simulink model "main"  (R2025a)
settings: Solver=FixedStepAuto  StartTime=0.0  StopTime=20  FixedStep=0.005  RelTol=1e-3
model workspace (MAT data in the model file):
  lowerLimit = 25
  speedMax = 10
  upperLimit = 75
libraries: simulink x5, simulink_extras x2
settings Model: PacingRate=0.100000  ParameterArgumentNames=speedMax  LastModifiedBy=alexc
settings SolverCC: ZeroCrossAlgorithm=Adaptive
settings OptimizationCC: BlockReduction=off  DefaultParameterBehavior=Inlined  BufferReuse=off
settings DebuggingCC: IgnoredZcDiagnostic=none
settings RTWCC: GPUComputeCapability=3.5

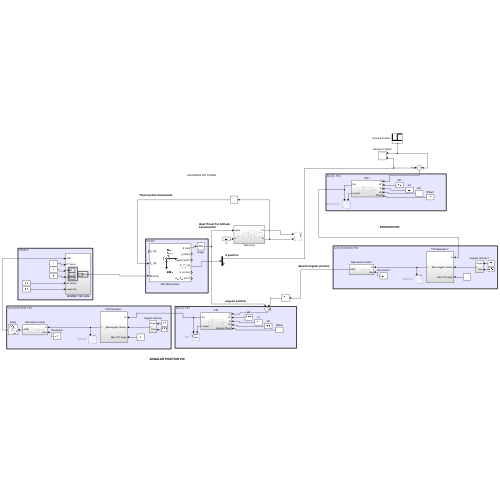
[thumbnail: Simulink's stored preview of the top-level diagram]
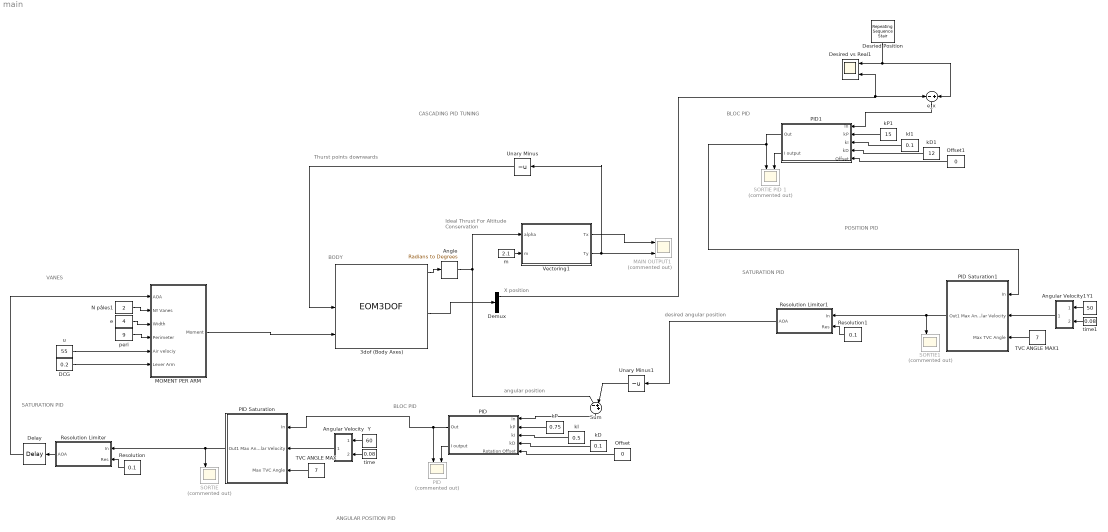
== system main ==
  note: CASCADING PID TUNING
  note: VANES
  note: SATURATION PID
  note: BODY
  note: BLOC PID
  note: BLOC PID
  note: SATURATION PID
  note: ANGULAR POSITION PID
  note: POSITION PID
  note: desired angular position
  note: angular position
  note: X position
  note: Ideal Thrust For Altitude Conservation
  note: Thurst points downwards
  3dof (Body Axes) : EOM3DOF  v_ini=0.0  mass=2.1  Iyy=0.038
  Angle : simulink_extras/Transformations/Radians to Degrees
  Angular Velocity : Subsystem
  Angular Velocity1 : Subsystem
  DCG : Constant  Value=0.2
  Delay : TransportDelay  DelayTime=0.005
  Demux : Demux  Outputs=2
  Desired vs Real1 : Scope  NumInputPorts=2
      settings: ActiveDisplayYMinimum=-0.47513093423326325  ActiveDisplayYMaximum=1.2413964602453749  DataLoggingVariableName=ScopeData5
  Desried Position : simulink/Sources/Repeating Sequence Stair  OutValues=[0,0.5]  tsamp=5  OutMin=[]  OutMax=[]  OutDataTypeStr=double  OutputDataTypeScalingMode=double  OutDataType=fixdt(0,8)  ConRadixGroup=Best Precision: Vector-wise  OutScaling=2^-12
  MAIN OUTPUT1 : Scope  Commented=on  NumInputPorts=2
      settings: ActiveDisplayYMinimum=-7.2954565061665075  ActiveDisplayYMaximum=8.1972905138472143
  MOMENT PER ARM : Subsystem
  N pâles1 : Constant  Value=2
  Offset : Constant  Value=0
  Offset1 : Constant  Value=0
  PID : Subsystem
  "PID " : Scope  Commented=on  NumInputPorts=2
      settings: ActiveDisplayYMinimum=-1  ActiveDisplayYMaximum=1  DataLoggingVariableName=ScopeData2
  PID Saturation : Subsystem
  PID Saturation1 : Subsystem
  PID1 : Subsystem
  Resolution : Constant  Value=0.1
  Resolution Limiter : Subsystem
  Resolution Limiter1 : Subsystem
  Resolution1 : Constant  Value=0.1
  SORTIE : Scope  Commented=on  NumInputPorts=2
      settings: ActiveDisplayYMinimum=-4.7113055005925766  ActiveDisplayYMaximum=4.7400570614554063  DataLoggingVariableName=ScopeData3
  SORTIE PID 1 : Scope  Commented=on  NumInputPorts=2
      settings: ActiveDisplayYMinimum=-12.890019352099706  ActiveDisplayYMaximum=16.05060564784133  DataLoggingVariableName=ScopeData4
  SORTIE1 : Scope  Commented=on  NumInputPorts=2
      settings: ActiveDisplayYMinimum=-6.75  ActiveDisplayYMaximum=0.75  DataLoggingVariableName=ScopeData6
  Sum : Sum  Inputs=|-++
  TVC ANGLE MAX : Constant  Value=7
  TVC ANGLE MAX1 : Constant  Value=7
  Unary Minus : UnaryMinus
  Unary Minus1 : UnaryMinus
  Vectoring1 : Subsystem
  Y : Constant  Value=60
  Y1 : Constant  Value=50
  e : Constant  Value=4
  e_x : Sum  Inputs=-+
  kD : Constant  Value=0.1
  kD1 : Constant  Value=12
  kI : Constant  Value=0.5
  kI1 : Constant  Value=0.1
  kP : Constant  Value=0.75
  kP1 : Constant  Value=15
  m : Constant  Value=2.1
  peri : Constant  Value=9
  time : Constant  Value=0.08
  time1 : Constant  Value=0.08
  u : Constant  Value=55
  wires:
  Angle/1 -> Sum/1, Vectoring1/1(alpha)
  3dof (Body Axes)/1 -> Angle/1
  N pâles1/1 -> MOMENT PER ARM/2(Nº Vanes)
  DCG/1 -> MOMENT PER ARM/6(Lever Arm)
  u/1 -> MOMENT PER ARM/5(Air velociy)
  e/1 -> MOMENT PER ARM/3(Width)
  peri/1 -> MOMENT PER ARM/4(Perimeter)
  Sum/1 -> PID/1(In)
  kP/1 -> PID/2(kP)
  kI/1 -> PID/3(kI)
  kD/1 -> PID/4(kD)
  Angular Velocity/1(Out1) -> PID Saturation/2(Max Angular Velocity)
  Y/1 -> Angular Velocity/1(Angle)
  time/1 -> Angular Velocity/2(Time)
  PID Saturation/1(Out1) -> Resolution Limiter/1(In), SORTIE/1
  Resolution/1 -> Resolution Limiter/2(Res)
  PID/1(Out) -> PID Saturation/1(In), "PID "/1
  TVC ANGLE MAX/1 -> PID Saturation/3(Max TVC Angle)
  Resolution Limiter/1(AOA) -> Delay/1
  Offset/1 -> PID/5(Rotation Offset)
  PID/2(I output) -> "PID "/2
  Delay/1 -> MOMENT PER ARM/1(AOA)
  MOMENT PER ARM/1(Moment) -> 3dof (Body Axes)/3
  m/1 -> Vectoring1/2(m)
  Vectoring1/2(Ty) -> Unary Minus/1, MAIN OUTPUT1/2
  Vectoring1/1(Tx) -> MAIN OUTPUT1/1
  3dof (Body Axes)/4 -> Demux/1
  Unary Minus/1 -> 3dof (Body Axes)/2
  Desried Position/1 -> e_x/2, Desired vs Real1/1
  PID1/2(I output) -> SORTIE PID 1/2
  e_x/1 -> PID1/1(In)
  kP1/1 -> PID1/2(kP)
  Offset1/1 -> PID1/5(Offset)
  kI1/1 -> PID1/3(kI)
  kD1/1 -> PID1/4(kD)
  time1/1 -> Angular Velocity1/2(Time)
  Y1/1 -> Angular Velocity1/1(Angle)
  PID1/1(Out) -> PID Saturation1/1(In), SORTIE PID 1/1
  TVC ANGLE MAX1/1 -> PID Saturation1/3(Max TVC Angle)
  PID Saturation1/1(Out1) -> Resolution Limiter1/1(In), SORTIE1/1
  Angular Velocity1/1(Out1) -> PID Saturation1/2(Max Angular Velocity)
  Resolution1/1 -> Resolution Limiter1/2(Res)
  Resolution Limiter1/1(AOA) -> Unary Minus1/1
  Demux/1 -> Desired vs Real1/2, e_x/1
  Unary Minus1/1 -> Sum/2

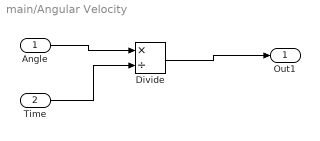
== system main/Angular Velocity ==
  Angle : Inport
  Time : Inport  Port=2
  Divide : Product  Inputs=*/
  Out1 : Outport
  wires:
  Time/1 -> Divide/2
  Angle/1 -> Divide/1
  Divide/1 -> Out1/1

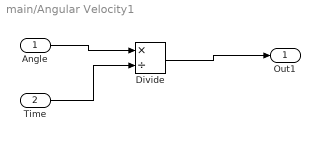
== system main/Angular Velocity1 ==
  Angle : Inport
  Time : Inport  Port=2
  Divide : Product  Inputs=*/
  Out1 : Outport
  wires:
  Time/1 -> Divide/2
  Angle/1 -> Divide/1
  Divide/1 -> Out1/1

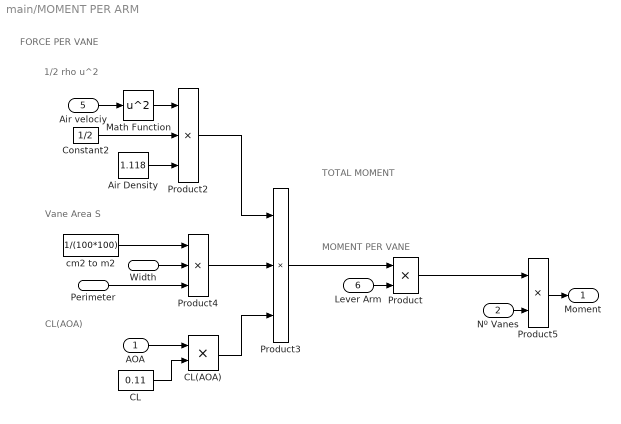
== system main/MOMENT PER ARM ==
  note: FORCE PER VANE
  note: CL(AOA)
  note: 1/2 rho u^2
  note: Vane Area S
  note: MOMENT PER VANE
  note: TOTAL MOMENT
  AOA : Inport
  Nº Vanes : Inport  Port=2
  Width : Inport  Port=3
  Perimeter : Inport  Port=4
  Air velociy : Inport  Port=5
  Lever Arm : Inport  Port=6
  Air Density : Constant  Value=1.118
  CL : Constant  Value=0.11
  CL(AOA) : Product
  Constant2 : Constant  Value=1/2
  Math Function : Math  Operator=square
  Product : Product
  Product2 : Product  Inputs=3
  Product3 : Product  Inputs=3
  Product4 : Product  Inputs=3
  Product5 : Product
  cm2 to m2 : Constant  Value=1/(100*100)
  Moment : Outport
  wires:
  Width/1 -> Product4/2
  Air velociy/1 -> Math Function/1
  cm2 to m2/1 -> Product4/1
  CL/1 -> CL(AOA)/2
  AOA/1 -> CL(AOA)/1
  Perimeter/1 -> Product4/3
  Lever Arm/1 -> Product/2
  Air Density/1 -> Product2/3
  Math Function/1 -> Product2/1
  Constant2/1 -> Product2/2
  Product/1 -> Product5/1
  Nº Vanes/1 -> Product5/2
  CL(AOA)/1 -> Product3/3
  Product4/1 -> Product3/2
  Product2/1 -> Product3/1
  Product3/1 -> Product/1
  Product5/1 -> Moment/1

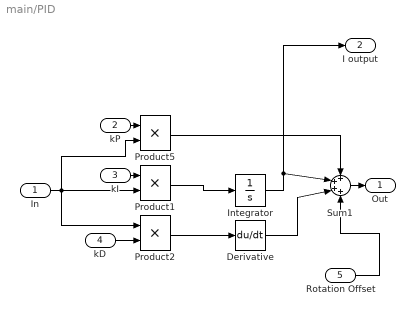
== system main/PID ==
  In : Inport
  kP : Inport  Port=2
  kI : Inport  Port=3
  kD : Inport  Port=4
  Rotation Offset : Inport  Port=5
  Derivative : Derivative
  Integrator : Integrator
  Product1 : Product
  Product2 : Product
  Product5 : Product
  Sum1 : Sum  Inputs=++++
  Out : Outport
  I output : Outport  Port=2
  wires:
  Product1/1 -> Integrator/1
  kD/1 -> Product2/2
  kI/1 -> Product1/1
  kP/1 -> Product5/1
  In/1 -> Product5/2, Product1/2, Product2/1
  Product2/1 -> Derivative/1
  Derivative/1 -> Sum1/3
  Integrator/1 -> I output/1, Sum1/2
  Product5/1 -> Sum1/1
  Sum1/1 -> Out/1
  Rotation Offset/1 -> Sum1/4

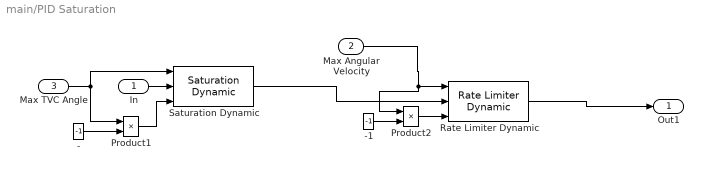
== system main/PID Saturation ==
  In : Inport
  Max Angular Velocity : Inport  Port=2
  Max TVC Angle : Inport  Port=3
  - : Constant  Value=-1
  -1 : Constant  Value=-1
  Product1 : Product
  Product2 : Product
  Rate Limiter Dynamic : simulink/Discontinuities/Rate Limiter Dynamic
  Saturation Dynamic : simulink/Discontinuities/Saturation Dynamic  OutMin=[]  OutMax=[]  OutDataTypeStr=Inherit: Same as second input  OutDataType=fixdt(1, 16)  OutScaling=2^-10  DoSatur=off
  Out1 : Outport
  wires:
  Max TVC Angle/1 -> Saturation Dynamic/1, Product1/1
  -/1 -> Product1/2
  In/1 -> Saturation Dynamic/2
  Product1/1 -> Saturation Dynamic/3
  Saturation Dynamic/1 -> Rate Limiter Dynamic/2
  Max Angular Velocity/1 -> Product2/1, Rate Limiter Dynamic/1
  -1/1 -> Product2/2
  Product2/1 -> Rate Limiter Dynamic/3
  Rate Limiter Dynamic/1 -> Out1/1

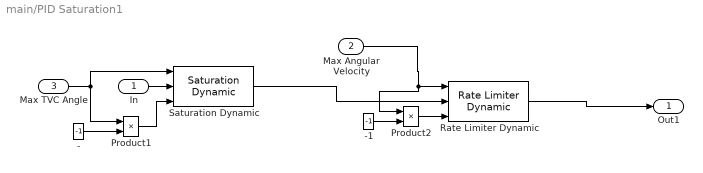
== system main/PID Saturation1 ==
  In : Inport
  Max Angular Velocity : Inport  Port=2
  Max TVC Angle : Inport  Port=3
  - : Constant  Value=-1
  -1 : Constant  Value=-1
  Product1 : Product
  Product2 : Product
  Rate Limiter Dynamic : simulink/Discontinuities/Rate Limiter Dynamic
  Saturation Dynamic : simulink/Discontinuities/Saturation Dynamic  OutMin=[]  OutMax=[]  OutDataTypeStr=Inherit: Same as second input  OutDataType=fixdt(1, 16)  OutScaling=2^-10  DoSatur=off
  Out1 : Outport
  wires:
  Max TVC Angle/1 -> Saturation Dynamic/1, Product1/1
  -/1 -> Product1/2
  In/1 -> Saturation Dynamic/2
  Product1/1 -> Saturation Dynamic/3
  Saturation Dynamic/1 -> Rate Limiter Dynamic/2
  Max Angular Velocity/1 -> Product2/1, Rate Limiter Dynamic/1
  -1/1 -> Product2/2
  Product2/1 -> Rate Limiter Dynamic/3
  Rate Limiter Dynamic/1 -> Out1/1

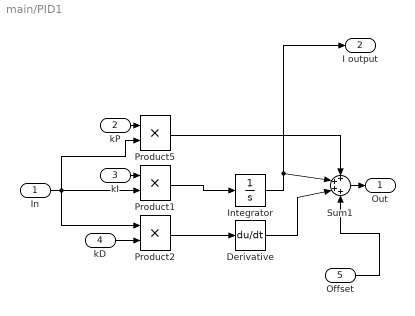
== system main/PID1 ==
  In : Inport
  kP : Inport  Port=2
  kI : Inport  Port=3
  kD : Inport  Port=4
  Offset : Inport  Port=5
  Derivative : Derivative
  Integrator : Integrator
  Product1 : Product
  Product2 : Product
  Product5 : Product
  Sum1 : Sum  Inputs=++++
  Out : Outport
  I output : Outport  Port=2
  wires:
  Product1/1 -> Integrator/1
  kD/1 -> Product2/2
  kI/1 -> Product1/1
  kP/1 -> Product5/1
  In/1 -> Product5/2, Product1/2, Product2/1
  Product2/1 -> Derivative/1
  Derivative/1 -> Sum1/3
  Integrator/1 -> I output/1, Sum1/2
  Product5/1 -> Sum1/1
  Sum1/1 -> Out/1
  Offset/1 -> Sum1/4

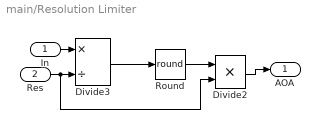
== system main/Resolution Limiter ==
  In : Inport
  Res : Inport  Port=2
  Divide2 : Product  Inputs=**
  Divide3 : Product  Inputs=*/
  Round : Rounding  Operator=round
  AOA : Outport
  wires:
  In/1 -> Divide3/1
  Res/1 -> Divide2/2, Divide3/2
  Divide3/1 -> Round/1
  Round/1 -> Divide2/1
  Divide2/1 -> AOA/1

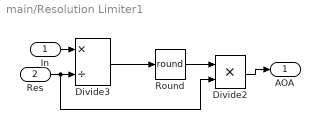
== system main/Resolution Limiter1 ==
  In : Inport
  Res : Inport  Port=2
  Divide2 : Product  Inputs=**
  Divide3 : Product  Inputs=*/
  Round : Rounding  Operator=round
  AOA : Outport
  wires:
  In/1 -> Divide3/1
  Res/1 -> Divide2/2, Divide3/2
  Divide3/1 -> Round/1
  Round/1 -> Divide2/1
  Divide2/1 -> AOA/1

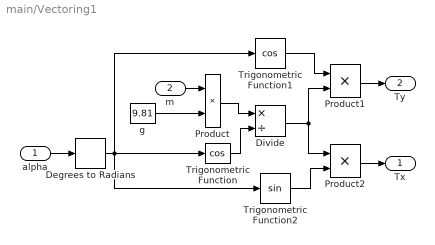
== system main/Vectoring1 ==
  alpha : Inport
  m : Inport  Port=2
  Degrees to Radians : simulink_extras/Transformations/Degrees to Radians
  Divide : Product  Inputs=*/
  Product : Product
  Product1 : Product
  Product2 : Product
  Trigonometric Function : Trigonometry  Operator=cos
  Trigonometric Function1 : Trigonometry  Operator=cos
  Trigonometric Function2 : Trigonometry
  g : Constant  Value=9.81
  Tx : Outport
  Ty : Outport  Port=2
  wires:
  m/1 -> Product/1
  g/1 -> Product/2
  alpha/1 -> Degrees to Radians/1
  Product2/1 -> Tx/1
  Product/1 -> Divide/1
  Trigonometric Function/1 -> Divide/2
  Degrees to Radians/1 -> Trigonometric Function2/1, Trigonometric Function1/1, Trigonometric Function/1
  Product1/1 -> Ty/1
  Trigonometric Function1/1 -> Product1/1
  Trigonometric Function2/1 -> Product2/2
  Divide/1 -> Product1/2, Product2/1
